simulink model "REG0LINEARIZOVANEsimulink"  (R2019b)
settings: Solver=FixedStepAuto  StartTime=0.0  StopTime=5  FixedStep=0.01  MaxStep=0.01  RelTol=1e-3
values from neighbouring files (symbols this model uses):
  x0 = [x10,x20,x30,x40]    [stavovaRovnice.m]
undefined symbols (not defined in the file or in its folder): Ar0, Br0, Cr0, Dr0, M_t
settings Model: Creator=jakub  LastModifiedBy=jakub

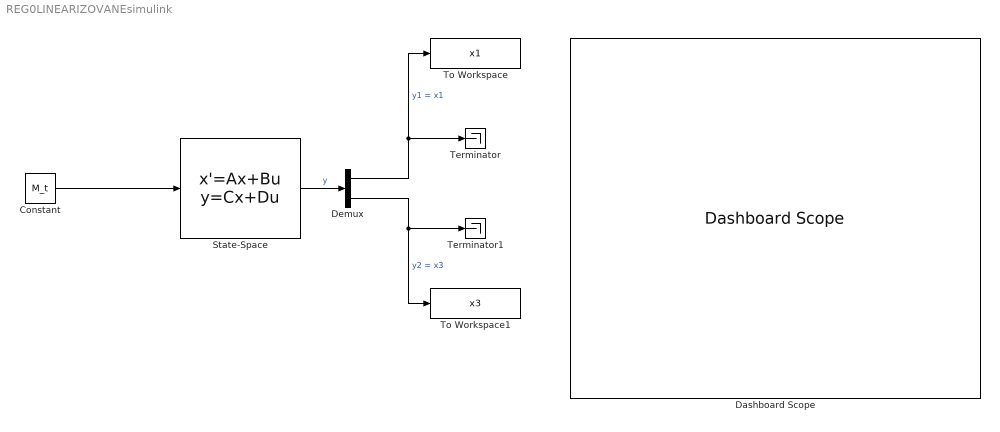
== system REG0LINEARIZOVANEsimulink ==
  Constant : Constant  Value=M_t
  Dashboard Scope : DashboardScope  Ymin=-1  Ymax=1
  Demux : Demux  Outputs=2
  State-Space : StateSpace  A=Ar0  B=Br0  C=Cr0  D=Dr0  InitialCondition=x0
  Terminator : Terminator
  Terminator1 : Terminator
  To Workspace : ToWorkspace  VariableName=x1  SaveFormat=Timeseries  SampleTime=-1
  To Workspace1 : ToWorkspace  VariableName=x3  SaveFormat=Timeseries  SampleTime=-1
  wires:
  Constant/1 -> State-Space/1
  State-Space/1 -> Demux/1  "y"
  Demux/1 -> To Workspace/1, Terminator/1  "y1 = x1"
  Demux/2 -> To Workspace1/1, Terminator1/1  "y2 = x3"
